simulink model "Suspension_Response_SIM"  (R2019a)
settings: Solver=VariableStepAuto  StartTime=0.0  StopTime=2.5  RelTol=1e-3
values from neighbouring files (symbols this model uses):
  r = 0.05    [Suspension_Response_UL.m]
  x1_equil = 0.7    [Suspension_Response_UL.m]
  x2_equil = 0.3    [Suspension_Response_UL.m]
undefined symbols (not defined in the file or in its folder): denG1, denG2, denG3, numG1, numG2, numG3
settings Model: Creator=Michael  LastModifiedBy=Michael

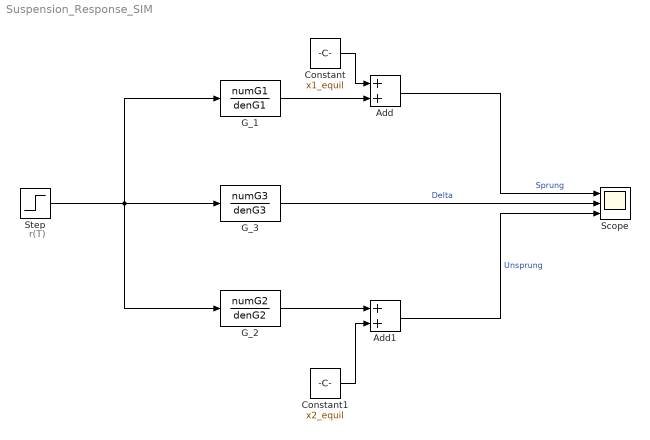
== system Suspension_Response_SIM ==
  note: r(T)
  Add : Sum
  Add1 : Sum
  Constant : Constant  Value=x1_equil
  Constant1 : Constant  Value=x2_equil
  G_1 : TransferFcn  Numerator=numG1  Denominator=denG1
  G_2 : TransferFcn  Numerator=numG2  Denominator=denG2
  G_3 : TransferFcn  Numerator=numG3  Denominator=denG3
  Scope : Scope  NumInputPorts=3
  Step : Step  Time=0  After=r  SampleTime=0
  wires:
  Step/1 -> G_2/1, G_3/1, G_1/1
  G_1/1 -> Add/2
  G_2/1 -> Add1/1
  G_3/1 -> Scope/2  "Delta"
  Constant/1 -> Add/1
  Add/1 -> Scope/1  "Sprung"
  Constant1/1 -> Add1/2
  Add1/1 -> Scope/3  "Unsprung"
